simulink model "sampleModel1412_2"  (R2023a)
settings: Solver=VariableStepAuto  StartTime=0.0  StopTime=10.0  RelTol=1e-3
libraries: hdlsllib x4, simulink x1
settings Model: Creator=user1  LastModifiedBy=user1

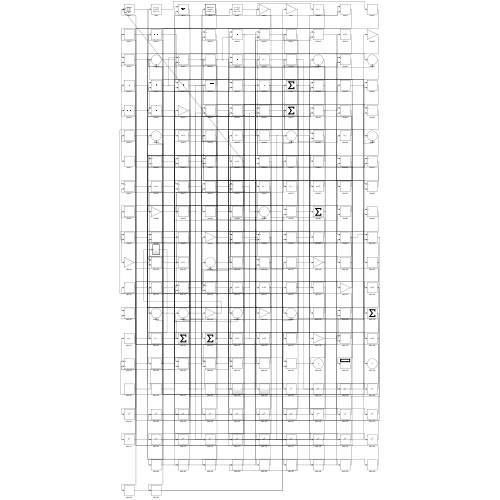
[thumbnail: Simulink's stored preview of the top-level diagram]
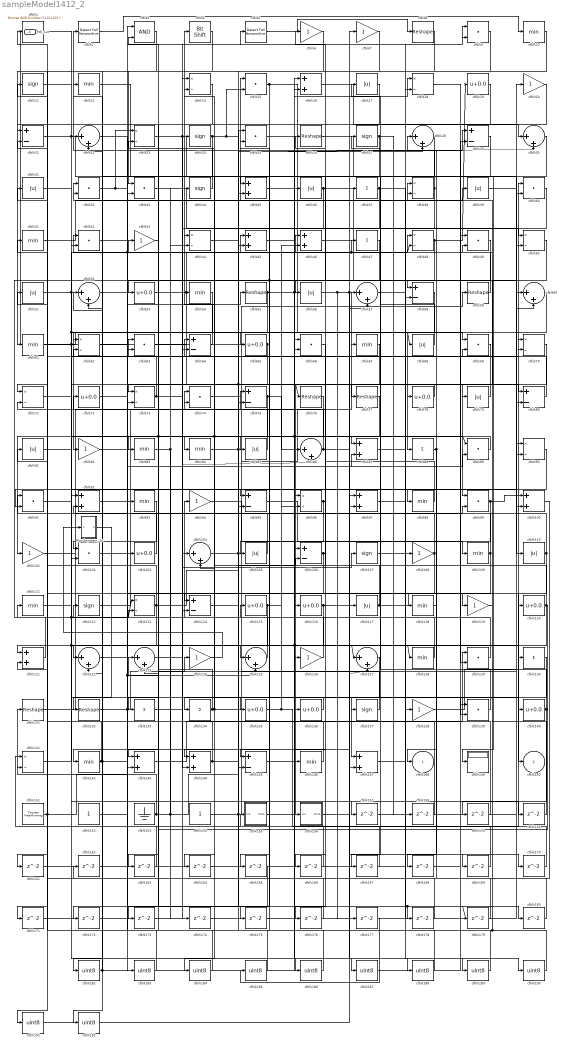
== system sampleModel1412_2 ==
  Mysubsystem_34 : Subsystem  TreatAsAtomicUnit=on  RTWFcnName=Mysubsystem_34
      settings: RTWFcnNameOpts=User specified  RTWFileNameOpts=Use function name
  cfblk1 : simulink/Logic and Bit Operations/Bitwise Operator  logicop=AND  UseBitMask=on  BitMask=bin2dec('11011001')  BitMaskRealWorld=Stored Integer
      settings: LibrarySourceBlock=|
      | hdlsllib/Logic and Bit
      | Operations/Bitwise
      | Operator
  cfblk{10,12,41,54,61,67,83..84,93,98,109,111,118,128,142,146} (16 alike) : MinMax  OutDataTypeStr=uint8
  cfblk{16,35,45..46,87,92,97,100,121,143..144,147} (12 alike) : Sum  OutDataTypeStr=uint8
  cfblk{6..7,20,43,82,94,101,108,119,124,126,138} (12 alike) : Gain  OutDataTypeStr=uint8
  cfblk{9,15,25,32..33,40,42,49,63,66,69,74,89,91,99,102,129,139} (18 alike) : DotProduct  OutDataTypeStr=uint8
  cfblk{19,53,65,72,78,103,115..116,120,135..136,140} (12 alike) : Bias  Bias=0.0  SaturateOnIntegerOverflow=off
  cfblk{22,28,30,52,57,60,86,104,122..123,125,127} (12 alike) : Sum  Inputs=|++  OutDataTypeStr=uint8
  cfblk{17,31,36,39,51,56,68,79,81,85,105,110,117} (13 alike) : Abs  OutDataTypeStr=uint8  SaturateOnIntegerOverflow=off
  cfblk{21,29,58,64,75,80,95,106,114,145} (10 alike) : Sum  Inputs=+-  OutDataTypeStr=uint8
  cfblk{11,24,27,34,107,112,137} (7 alike) : Signum
  cfblk{14,18,23,38,44,48,50,62,70..71,73,90,96,113,141} (15 alike) : Product  Inputs=*/  OutDataTypeStr=uint8  RndMeth=Zero  SaturateOnIntegerOverflow=on
  cfblk{37,47,88,130,133..134} (6 alike) : Sum  Inputs=+  OutDataTypeStr=uint8
  cfblk{8,26,55,59,76..77,131..132} (8 alike) : Reshape
  cfblk149 : Display
  cfblk151 : hdlsllib/Sources/Counter Free-Running  NumBits=16  tsamp=-1
  cfblk152 : Constant  OutDataTypeStr=uint8  SampleTime=-1
  cfblk153 : Ground
  cfblk154 : Constant  OutDataTypeStr=uint8  SampleTime=-1
  cfblk155 : Subsystem
      settings: LibrarySourceBlock=|
      | hdlsllib/Ports &
      | Subsystems/Subsystem
  cfblk156 : Subsystem
      settings: LibrarySourceBlock=|
      | hdlsllib/Ports &
      | Subsystems/Subsystem
  cfblk{157..180} (24 alike) : Delay  SampleTime=1
  cfblk{182..192} (11 alike) : DataTypeConversion  OutDataTypeStr=uint8  SaturateOnIntegerOverflow=off  RndMeth=Floor
  cfblk2 : hdlsllib/Logic and Bit Operations/Detect Fall Nonpositive  vinit=0  OutDataTypeStr=uint8
  cfblk3 : Logic  AllPortsSameDT=off  OutDataTypeStr=boolean
  cfblk4 : hdlsllib/Logic and Bit Operations/Bit Shift  mode=Shift Left Logical  N=0
  cfblk5 : hdlsllib/Logic and Bit Operations/Detect Fall Nonpositive  vinit=0  OutDataTypeStr=uint8
  cfblk148 : Outport  OutDataTypeStr=uint8  VectorParamsAs1DForOutWhenUnconnected=off
  cfblk150 : Outport  Port=2  OutDataTypeStr=uint8  VectorParamsAs1DForOutWhenUnconnected=off
  Hdl_out : Outport  Port=3  OutDataTypeStr=uint8
  wires:
  cfblk131/1 -> cfblk74/1
  cfblk53/1 -> cfblk99/1, cfblk7/1
  cfblk63/1 -> cfblk156/1(In1)
  cfblk119/1 -> cfblk32/1
  cfblk153/1 -> cfblk34/1, cfblk35/2, cfblk131/1
  cfblk125/1 -> cfblk112/1
  cfblk75/1 -> cfblk101/1, cfblk86/1
  cfblk121/1 -> cfblk58/1
  cfblk23/1 -> cfblk149/1, cfblk86/2, cfblk9/2
  cfblk135/1 -> cfblk40/1, cfblk96/2
  cfblk7/1 -> cfblk33/1
  cfblk48/1 -> cfblk19/1, cfblk63/2
  cfblk41/1 -> cfblk15/1
  cfblk120/1 -> cfblk142/1, cfblk23/2, cfblk175/1
  cfblk5/1 -> cfblk8/1
  cfblk96/1 -> cfblk145/1, cfblk166/1
  cfblk154/1 -> cfblk59/1, cfblk106/2
  cfblk76/1 -> cfblk163/1, cfblk164/1
  cfblk98/1 -> cfblk74/2
  cfblk136/1 -> cfblk134/1
  cfblk37/1 -> cfblk138/1, cfblk95/1
  cfblk68/1 -> cfblk42/1
  cfblk117/1 -> cfblk119/1, cfblk26/1
  cfblk143/1 -> cfblk129/1
  cfblk19/1 -> cfblk53/1
  cfblk60/1 -> cfblk82/1
  cfblk33/1 -> cfblk50/1
  cfblk34/1 -> cfblk4/1
  cfblk138/1 -> cfblk20/1
  cfblk97/1 -> cfblk190/1
  cfblk130/1 -> cfblk147/1
  cfblk38/1 -> cfblk2/1, cfblk114/1
  cfblk61/1 -> cfblk65/1, cfblk96/1
  cfblk15/1 -> cfblk88/1, cfblk105/1
  cfblk146/1 -> cfblk91/1
  cfblk21/1 -> cfblk64/2, cfblk80/2, cfblk35/1
  cfblk115/1 -> cfblk122/1, cfblk46/2
  cfblk102/1 -> cfblk99/2
  cfblk108/1 -> cfblk64/1, cfblk137/1
  cfblk109/1 -> cfblk17/1, cfblk191/1
  cfblk94/1 -> cfblk106/1
  cfblk84/1 -> cfblk57/1, cfblk30/2
  cfblk55/1 -> cfblk69/1, cfblk18/1, cfblk114/2
  cfblk78/1 -> cfblk73/1
  cfblk56/1 -> cfblk29/1, cfblk127/2, cfblk177/1
  cfblk83/1 -> cfblk44/2, cfblk174/1
  cfblk132/1 -> cfblk125/2, cfblk48/1, cfblk124/1
  cfblk112/1 -> cfblk16/1
  cfblk123/1 -> cfblk45/1
  cfblk29/1 -> cfblk62/1
  cfblk106/1 -> cfblk6/1, cfblk171/1
  cfblk86/1 -> cfblk51/1, cfblk170/1
  cfblk72/1 -> cfblk5/1
  cfblk152/1 -> cfblk93/1
  cfblk47/1 -> cfblk85/1, cfblk145/2
  cfblk69/1 -> cfblk143/1
  cfblk111/1 -> cfblk46/1
  cfblk142/1 -> cfblk12/1, cfblk89/2, cfblk81/1
  cfblk155/1(Out1) -> cfblk38/1
  cfblk81/1 -> cfblk87/1
  cfblk122/1 -> cfblk55/1
  cfblk54/1 -> cfblk143/2
  cfblk24/1 -> cfblk15/2, cfblk28/2, cfblk73/2
  cfblk36/1 -> cfblk129/2, cfblk144/2
  cfblk133/1 -> cfblk107/1
  cfblk110/1 -> cfblk150/1, cfblk14/2
  cfblk4/1 -> cfblk61/1
  cfblk90/1 -> cfblk91/2
  cfblk66/1 -> cfblk136/1
  cfblk49/1 -> cfblk144/1
  cfblk10/1 -> cfblk71/1
  cfblk12/1 -> cfblk60/1
  cfblk58/1 -> cfblk123/2
  cfblk74/1 -> cfblk37/1
  cfblk140/1 -> cfblk115/1, cfblk159/1
  cfblk26/1 -> cfblk40/2
  cfblk87/1 -> cfblk108/1
  cfblk156/1(Out1) -> cfblk117/1
  cfblk44/1 -> cfblk76/1, cfblk98/1
  cfblk27/1 -> cfblk104/2, cfblk158/1
  cfblk145/1 -> cfblk36/1
  cfblk39/1 -> cfblk110/1
  cfblk18/1 -> cfblk80/1
  cfblk144/1 -> cfblk22/1, cfblk70/1
  cfblk141/1 -> cfblk113/1, cfblk70/2
  cfblk104/1 -> cfblk67/1, cfblk87/2
  cfblk17/1 -> cfblk42/2
  cfblk57/1 -> cfblk109/1
  cfblk28/1 -> cfblk56/1
  cfblk2/1 -> cfblk10/1
  cfblk14/1 -> cfblk21/1
  cfblk77/1 -> cfblk133/1, cfblk102/2
  cfblk114/1 -> cfblk178/1, cfblk179/1
  cfblk85/1 -> cfblk75/1
  cfblk82/1 -> cfblk16/2
  cfblk101/1 -> cfblk33/2
  cfblk116/1 -> cfblk125/1, cfblk189/1
  cfblk113/1 -> cfblk121/1, cfblk11/1, cfblk95/2
  cfblk46/1 -> cfblk60/2
  cfblk80/1 -> cfblk41/1
  cfblk99/1 -> cfblk146/1, cfblk100/1
  cfblk139/1 -> cfblk27/1
  cfblk134/1 -> cfblk90/2, cfblk54/1, cfblk92/2
  cfblk137/1 -> cfblk32/2
  cfblk95/1 -> cfblk118/1
  cfblk32/1 -> cfblk147/2, cfblk23/1
  cfblk59/1 -> cfblk24/1
  cfblk126/1 -> cfblk94/1
  cfblk79/1 -> cfblk78/1
  cfblk8/1 -> cfblk75/2
  cfblk93/1 -> cfblk102/1
  cfblk92/1 -> cfblk47/1, cfblk48/2, cfblk39/1
  cfblk50/1 -> cfblk79/1
  cfblk103/1 -> cfblk21/2
  cfblk89/1 -> cfblk83/1
  cfblk52/1 -> cfblk120/1
  cfblk129/1 -> cfblk22/2
  cfblk64/1 -> cfblk44/1
  cfblk3/1 -> cfblk182/1
  cfblk16/1 -> cfblk30/1
  cfblk11/1 -> cfblk68/1, cfblk130/1
  cfblk71/1 -> cfblk140/1
  cfblk73/1 -> cfblk52/2, cfblk100/2
  cfblk20/1 -> cfblk135/1
  cfblk35/1 -> cfblk139/2, cfblk128/1, cfblk89/1
  cfblk107/1 -> cfblk9/1
  cfblk88/1 -> cfblk148/1, cfblk28/1
  cfblk30/1 -> cfblk77/1
  cfblk67/1 -> cfblk84/1
  cfblk151/1 -> cfblk103/1, cfblk31/1
  cfblk45/1 -> cfblk66/2
  cfblk105/1 -> cfblk63/1
  cfblk128/1 -> cfblk111/1
  cfblk51/1 -> cfblk126/1, cfblk43/1
  cfblk31/1 -> cfblk127/1, cfblk188/1
  cfblk91/1 -> cfblk157/1
  cfblk157/1 -> cfblk90/1
  cfblk158/1 -> cfblk92/1
  cfblk159/1 -> cfblk71/2
  cfblk22/1 -> cfblk160/1
  cfblk160/1 -> cfblk69/2
  cfblk9/1 -> cfblk161/1
  cfblk161/1 -> cfblk45/2
  cfblk100/1 -> cfblk162/1
  cfblk162/1 -> cfblk14/1
  cfblk163/1 -> cfblk141/1
  cfblk164/1 -> cfblk18/2
  cfblk40/1 -> cfblk165/1
  cfblk166/1 -> cfblk123/1
  cfblk70/1 -> cfblk167/1
  cfblk167/1 -> cfblk52/1
  cfblk118/1 -> cfblk168/1
  cfblk168/1 -> cfblk29/2
  cfblk147/1 -> cfblk169/1
  cfblk169/1 -> cfblk62/2
  cfblk170/1 -> cfblk122/2
  cfblk171/1 -> cfblk50/2
  cfblk6/1 -> cfblk172/1
  cfblk172/1 -> cfblk104/1
  cfblk43/1 -> cfblk173/1
  cfblk173/1 -> cfblk58/2
  cfblk174/1 -> cfblk139/1
  cfblk175/1 -> cfblk57/2
  cfblk127/1 -> cfblk176/1
  cfblk176/1 -> cfblk66/1
  cfblk178/1 -> cfblk113/2
  cfblk179/1 -> cfblk38/2
  cfblk42/1 -> cfblk180/1
  cfblk180/1 -> cfblk121/2
  cfblk182/1 -> cfblk116/1, cfblk72/1
  cfblk62/1 -> cfblk183/1
  cfblk183/1 -> cfblk3/1
  cfblk65/1 -> cfblk184/1, Hdl_out/1
  cfblk184/1 -> cfblk3/2
  cfblk177/1 -> cfblk185/1
  cfblk185/1 -> cfblk1/1
  cfblk1/1 -> cfblk186/1
  cfblk186/1 -> cfblk141/2
  cfblk25/1 -> cfblk187/1
  cfblk187/1 -> cfblk49/1
  cfblk188/1 -> cfblk25/1
  cfblk189/1 -> cfblk25/2
  cfblk190/1 -> cfblk49/2, cfblk155/1(In1)
  cfblk191/1 -> cfblk97/1
  cfblk165/1 -> cfblk192/1
  cfblk192/1 -> cfblk97/2
  cfblk124/1 -> Mysubsystem_34/1(In1)
  Mysubsystem_34/1(Out1) -> cfblk132/1

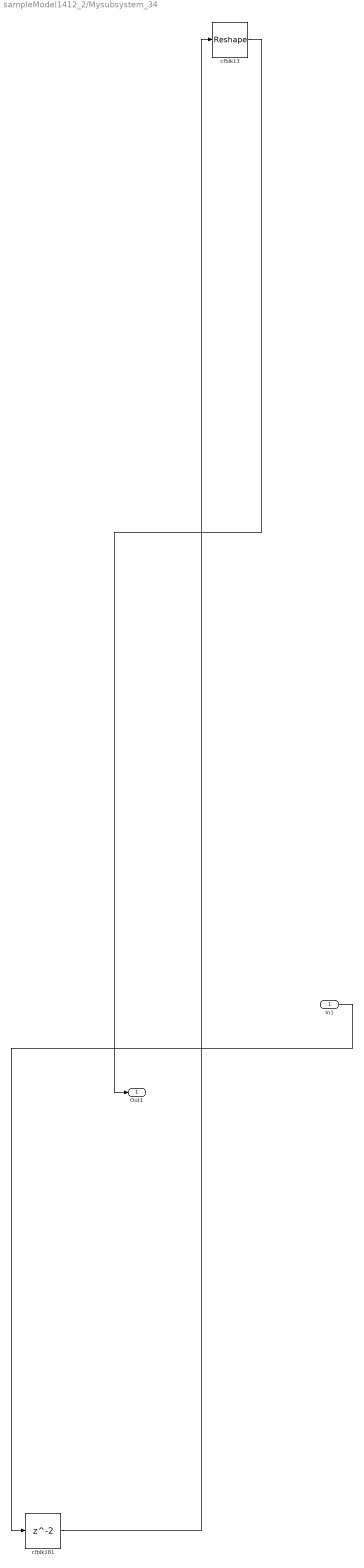
== system sampleModel1412_2/Mysubsystem_34 ==
  In1 : Inport
  cfblk13 : Reshape
  cfblk181 : Delay  SampleTime=1
  Out1 : Outport
  wires:
  cfblk13/1 -> Out1/1
  cfblk181/1 -> cfblk13/1
  In1/1 -> cfblk181/1

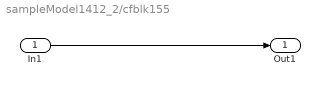
== system sampleModel1412_2/cfblk155 ==
  In1 : Inport
  Out1 : Outport
  wires:
  In1/1 -> Out1/1

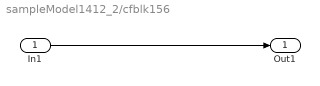
== system sampleModel1412_2/cfblk156 ==
  In1 : Inport
  Out1 : Outport
  wires:
  In1/1 -> Out1/1
